simulink model "rtwdemo_eMLcallsC"  (Simulink 7.2)
settings: Solver=FixedStepDiscrete  StartTime=0.0  StopTime=10.0  RelTol=1e-3
settings Model: Creator=ajayaram  LastModifiedBy=ajayaram
settings OptimizationCC: InitFltsAndDblsToZero=on  EfficientMapNaN2IntZero=off  OptimizeModelRefInitCode=on  LifeSpan=1
settings SFSimCC: SimCustomHeaderCode="#include \"add.h\""  SimUserSources=add.c
settings RTWCC: SystemTargetFile=ert.tlc  TemplateMakefile=ert_default_tmf  Description=Real-Time Workshop Embedded Coder (no auto configuration)  GenerateReport=on  ProcessScript=ert_make_rtw_hook  CustomHeaderCode="#include \"add.h\""  CustomSource=add.c  IncludeHyperlinkInReport=on  LaunchReport=on
settings CodeAppCC: IgnoreCustomStorageClasses=off
settings ERTTargetCC: GenerateSampleERTMain=on  InlinedParameterPlacement=NonHierarchical  ERTCustomFileTemplate=example_file_process.tlc

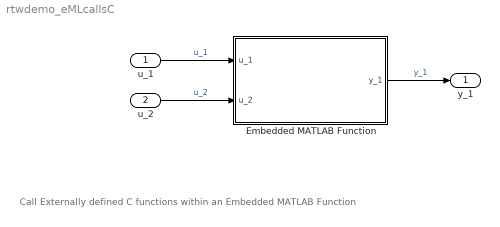
== system rtwdemo_eMLcallsC ==
  note: Call Externally defined C functions
      | within an Embedded MATLAB Function
  u_1 : Inport  OutDataType=sfix(16)  OutScaling=2^0
  u_2 : Inport  Port=2  OutDataType=sfix(16)  OutScaling=2^0
  Embedded MATLAB Function : Stateflow chart
  y_1 : Outport  OutDataType=sfix(16)  OutScaling=2^0
  wires:
  u_1/1 -> Embedded MATLAB Function/1(u_1)  "u_1"
  Embedded MATLAB Function/1(y_1) -> y_1/1  "y_1"
  u_2/1 -> Embedded MATLAB Function/2(u_2)  "u_2"

== matlab function Embedded MATLAB Function ==
  data: u_1 input double; y_1 output double; u_2 input double

function y_1 = eMLadder(u_1, u_2)

%Set the class and size of output
y_1 = u_1; 

%Call external C function
y_1 = eml.ceval('add',u_1,u_2);

end
